simulink model "Queueing_system"  (R2023b)
settings: Solver=VariableStepAuto  StartTime=0.0  StopTime=100000.0  RelTol=1e-3
values from neighbouring files (symbols this model uses):
  m = 20    [Lab2_driver.m]
undefined symbols (not defined in the file or in its folder): entity, entitySys, n, ShowAttrib
settings Model: Creator=alberto  LastModifiedBy=alberto

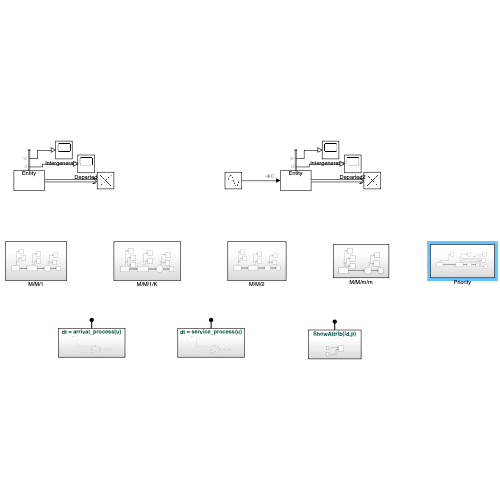
[thumbnail: Simulink's stored preview of the top-level diagram]
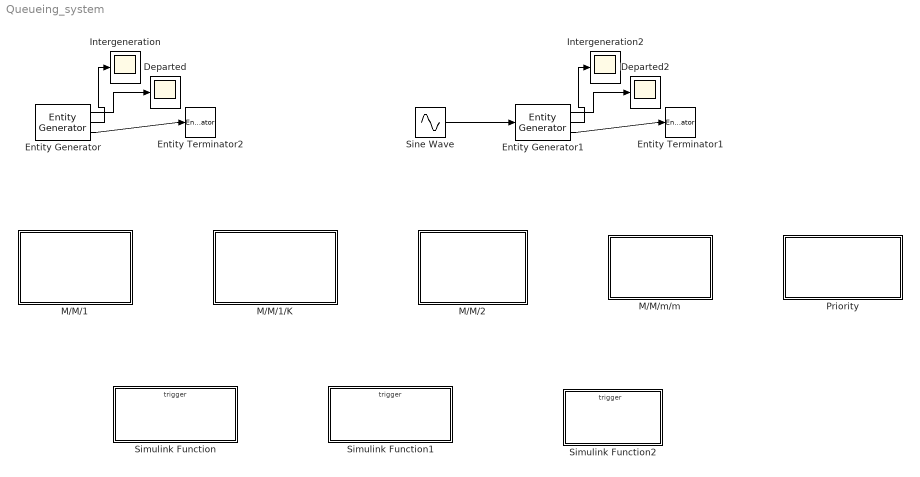
== system Queueing_system ==
  Departed : Scope
  Departed2 : Scope
  Entity Generator : EntityGenerator  OutputPortMessageModes=n,n,m  Period=0.5  IntergenerationTimeAction=dt = arrival_process(1/mG);  GenerateEntityAtSimulationStart=off  NumberEntitiesDeparted=on  AverageIntergenerationTime=on  EntityType=Structured  EntityTypeName=Entity
      settings: OutputPortMap=o0,o2,o3
  Entity Generator1 : EntityGenerator  OutputPortMessageModes=n,n,m  TimeSource=Signal port  Period=0.5  IntergenerationTimeAction=dt = arrival_process(1/mG);  GenerateEntityAtSimulationStart=off  NumberEntitiesDeparted=on  AverageIntergenerationTime=on  EntityType=Structured  EntityTypeName=Entity
      settings: InputPortMap=u1  OutputPortMap=o0,o2,o3
  Entity Terminator1 : EntityTerminator  InputPortMessageModes=m
  Entity Terminator2 : EntityTerminator  InputPortMessageModes=m
  Intergeneration : Scope
  Intergeneration2 : Scope
  M/M/1 : Subsystem
  M/M/1/K : Subsystem
  M/M/2 : Subsystem
  M/M/m/m : Subsystem
  Priority : Subsystem
  Simulink Function : Subsystem  TreatAsAtomicUnit=on
  Simulink Function1 : Subsystem  TreatAsAtomicUnit=on
  Simulink Function2 : Subsystem  TreatAsAtomicUnit=on
  Sine Wave : Sin  Bias=1.5  Frequency=2*pi  SampleTime=0
  wires:
  Sine Wave/1 -> Entity Generator1/1
  Entity Generator1/3 -> Entity Terminator1/1
  Entity Generator/3 -> Entity Terminator2/1
  Entity Generator/2 -> Intergeneration/1
  Entity Generator/1 -> Departed/1
  Entity Generator1/1 -> Departed2/1
  Entity Generator1/2 -> Intergeneration2/1

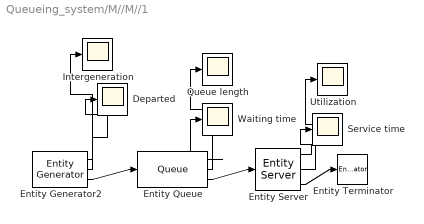
== system Queueing_system/M//M//1 ==
  Departed : Scope
  Entity Generator2 : EntityGenerator  OutputPortMessageModes=n,n,m  TimeSource=MATLAB action  Period=0.5  IntergenerationTimeAction=dt = arrival_process(1/mG);  GenerateEntityAtSimulationStart=off  NumberEntitiesDeparted=on  AverageIntergenerationTime=on  EntityType=Structured  EntityTypeName=Entity
      settings: OutputPortMap=o0,o2,o3
  Entity Queue : Queue  InputPortMessageModes=m  OutputPortMessageModes=n,n,m  Capacity=Inf  AverageWait=on  AverageQueueLength=on
      settings: OutputPortMap=o2,o3,o5
  Entity Server : EntityServer  InputPortMessageModes=m  OutputPortMessageModes=n,n,m  Capacity=1  ServiceTimeSource=MATLAB action  ServiceTimeAction=dt = service_process(1/mS);  AverageWait=on  Utilization=on
      settings: OutputPortMap=o4,o5,o9
  Entity Terminator : EntityTerminator  InputPortMessageModes=m
  Intergeneration : Scope
  Queue length : Scope
  Service time : Scope
  Utilization : Scope
  Waiting time : Scope
  wires:
  Entity Queue/1 -> Waiting time/1
  Entity Generator2/2 -> Intergeneration/1
  Entity Queue/3 -> Entity Server/1
  Entity Server/1 -> Service time/1
  Entity Generator2/3 -> Entity Queue/1
  Entity Server/2 -> Utilization/1
  Entity Generator2/1 -> Departed/1
  Entity Server/3 -> Entity Terminator/1
  Entity Queue/2 -> Queue length/1

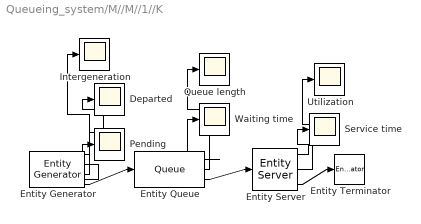
== system Queueing_system/M//M//1//K ==
  Departed : Scope
  Entity Generator : EntityGenerator  OutputPortMessageModes=n,n,n,m  TimeSource=MATLAB action  Period=0.5  IntergenerationTimeAction=dt = arrival_process(1/mG);  GenerateEntityAtSimulationStart=off  NumberEntitiesDeparted=on  PendingEntityInBlock=on  AverageIntergenerationTime=on  EntityType=Structured  EntityTypeName=Entity
      settings: OutputPortMap=o0,o1,o2,o3
  Entity Queue : Queue  InputPortMessageModes=m  OutputPortMessageModes=n,n,m  Capacity=K  AverageWait=on  AverageQueueLength=on
      settings: OutputPortMap=o2,o3,o5
  Entity Server : EntityServer  InputPortMessageModes=m  OutputPortMessageModes=n,n,m  Capacity=1  ServiceTimeSource=MATLAB action  ServiceTimeAction=dt = service_process(1/mS);  AverageWait=on  Utilization=on
      settings: OutputPortMap=o4,o5,o9
  Entity Terminator : EntityTerminator  InputPortMessageModes=m
  Intergeneration : Scope
  Pending : Scope
  Queue length : Scope
  Service time : Scope
  Utilization : Scope
  Waiting time : Scope
  wires:
  Entity Server/2 -> Utilization/1
  Entity Queue/2 -> Queue length/1
  Entity Queue/1 -> Waiting time/1
  Entity Queue/3 -> Entity Server/1
  Entity Generator/4 -> Entity Queue/1
  Entity Generator/3 -> Intergeneration/1
  Entity Generator/1 -> Departed/1
  Entity Generator/2 -> Pending/1
  Entity Server/1 -> Service time/1
  Entity Server/3 -> Entity Terminator/1

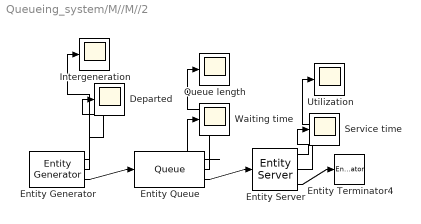
== system Queueing_system/M//M//2 ==
  Departed : Scope
  Entity Generator : EntityGenerator  OutputPortMessageModes=n,n,m  TimeSource=MATLAB action  Period=0.5  IntergenerationTimeAction=dt = arrival_process(1/mG);  GenerateEntityAtSimulationStart=off  NumberEntitiesDeparted=on  AverageIntergenerationTime=on  EntityType=Structured  EntityTypeName=Entity
      settings: OutputPortMap=o0,o2,o3
  Entity Queue : Queue  InputPortMessageModes=m  OutputPortMessageModes=n,n,m  Capacity=Inf  AverageWait=on  AverageQueueLength=on
      settings: OutputPortMap=o2,o3,o5
  Entity Server : EntityServer  InputPortMessageModes=m  OutputPortMessageModes=n,n,m  Capacity=2  ServiceTimeSource=MATLAB action  ServiceTimeAction=dt = service_process(1/mS);  AverageWait=on  Utilization=on
      settings: OutputPortMap=o4,o5,o9
  Entity Terminator4 : EntityTerminator  InputPortMessageModes=m
  Intergeneration : Scope
  Queue length : Scope
  Service time : Scope
  Utilization : Scope
  Waiting time : Scope
  wires:
  Entity Generator/2 -> Intergeneration/1
  Entity Queue/1 -> Waiting time/1
  Entity Server/1 -> Service time/1
  Entity Server/3 -> Entity Terminator4/1
  Entity Queue/2 -> Queue length/1
  Entity Queue/3 -> Entity Server/1
  Entity Server/2 -> Utilization/1
  Entity Generator/1 -> Departed/1
  Entity Generator/3 -> Entity Queue/1

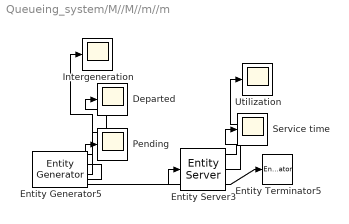
== system Queueing_system/M//M//m//m ==
  Departed : Scope
  Entity Generator5 : EntityGenerator  OutputPortMessageModes=n,n,n,m  TimeSource=MATLAB action  Period=0.5  IntergenerationTimeAction=dt = arrival_process(1/mG);  GenerateEntityAtSimulationStart=off  NumberEntitiesDeparted=on  PendingEntityInBlock=on  AverageIntergenerationTime=on  EntityType=Structured  EntityTypeName=Entity
      settings: OutputPortMap=o0,o1,o2,o3
  Entity Server3 : EntityServer  InputPortMessageModes=m  OutputPortMessageModes=n,n,m  Capacity=m  ServiceTimeSource=MATLAB action  ServiceTimeAction=dt = service_process(1/mS);  AverageWait=on  Utilization=on
      settings: OutputPortMap=o4,o5,o9
  Entity Terminator5 : EntityTerminator  InputPortMessageModes=m
  Intergeneration : Scope
  Pending : Scope
  Service time : Scope
  Utilization : Scope
  wires:
  Entity Generator5/3 -> Intergeneration/1
  Entity Server3/2 -> Utilization/1
  Entity Server3/1 -> Service time/1
  Entity Server3/3 -> Entity Terminator5/1
  Entity Generator5/2 -> Pending/1
  Entity Generator5/4 -> Entity Server3/1
  Entity Generator5/1 -> Departed/1

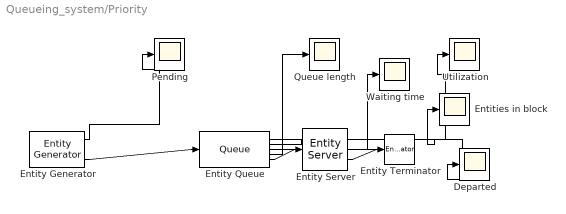
== system Queueing_system/Priority ==
  Departed : Scope
  Entities in block : Scope
  Entity Generator : EntityGenerator  OutputPortMessageModes=n,m  TimeSource=MATLAB action  Period=8  IntergenerationTimeAction=dt = arrival_process(1.5/mG);  GenerateEntityAtSimulationStart=off  GenerateAction=entity.MyPriority = randi(2);  AttributeName=MyPriority  AttributeInitialValue=0  PendingEntityInBlock=on  EntityType=Structured  EntityTypeName=Entity_p
      settings: OutputPortMap=o1,o3
  Entity Queue : Queue  InputPortMessageModes=m  OutputPortMessageModes=n,n,n,n,m  Capacity=Inf  QueueType=Priority  PrioritySource=MyPriority  ExitAction=ShowAttrib(entitySys.id, entity.MyPriority);  NumberEntitiesDeparted=on  NumberEntitiesInBlock=on  AverageWait=on  AverageQueueLength=on
      settings: OutputPortMap=o0,o1,o2,o3,o5
  Entity Server : EntityServer  InputPortMessageModes=m  OutputPortMessageModes=n,m  Capacity=1  ServiceTimeSource=MATLAB action  ServiceTimeAction=dt = service_process(1/mS);  Utilization=on
      settings: OutputPortMap=o5,o9
  Entity Terminator : EntityTerminator  InputPortMessageModes=m
  Pending : Scope
  Queue length : Scope
  Utilization : Scope
  Waiting time : Scope
  wires:
  Entity Queue/4 -> Queue length/1
  Entity Server/2 -> Entity Terminator/1
  Entity Generator/2 -> Entity Queue/1
  Entity Server/1 -> Utilization/1
  Entity Queue/1 -> Departed/1
  Entity Generator/1 -> Pending/1
  Entity Queue/5 -> Entity Server/1
  Entity Queue/3 -> Waiting time/1
  Entity Queue/2 -> Entities in block/1

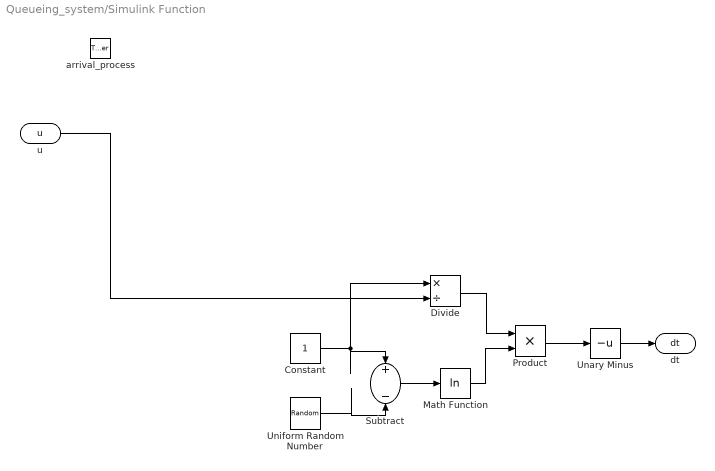
== system Queueing_system/Simulink Function ==
  arrival_process : TriggerPort  TriggerType=function-call  IsSimulinkFunction=on  FunctionName=arrival_process  FunctionVisibility=scoped  VariantControl=(inherit)
  Constant : Constant
  Divide : Product  Inputs=*/
  Math Function : Math  Operator=log
  Product : Product
  Subtract : Sum  Inputs=+-
  Unary Minus : UnaryMinus
  Uniform Random Number : UniformRandomNumber  Minimum=0  Seed=randi(3333333)
  u : ArgIn  DisableCoverage=on  ArgumentName=u
  dt : ArgOut  DisableCoverage=on  ArgumentName=dt
  wires:
  Product/1 -> Unary Minus/1
  Constant/1 -> Divide/1, Subtract/1
  u/1 -> Divide/2
  Uniform Random Number/1 -> Subtract/2
  Divide/1 -> Product/1
  Math Function/1 -> Product/2
  Subtract/1 -> Math Function/1
  Unary Minus/1 -> dt/1

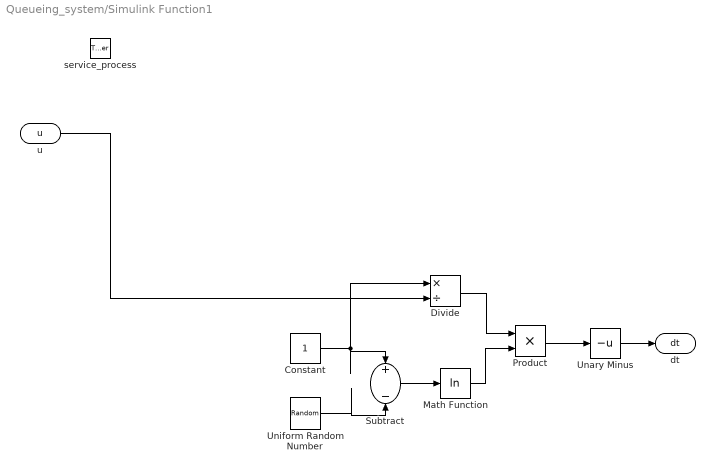
== system Queueing_system/Simulink Function1 ==
  service_process : TriggerPort  TriggerType=function-call  IsSimulinkFunction=on  FunctionName=service_process  FunctionVisibility=scoped  VariantControl=(inherit)
  Constant : Constant
  Divide : Product  Inputs=*/
  Math Function : Math  Operator=log
  Product : Product
  Subtract : Sum  Inputs=+-
  Unary Minus : UnaryMinus
  Uniform Random Number : UniformRandomNumber  Minimum=0  Seed=randi(7583)
  u : ArgIn  DisableCoverage=on  ArgumentName=u
  dt : ArgOut  DisableCoverage=on  ArgumentName=dt
  wires:
  Product/1 -> Unary Minus/1
  Constant/1 -> Divide/1, Subtract/1
  u/1 -> Divide/2
  Uniform Random Number/1 -> Subtract/2
  Divide/1 -> Product/1
  Math Function/1 -> Product/2
  Subtract/1 -> Math Function/1
  Unary Minus/1 -> dt/1

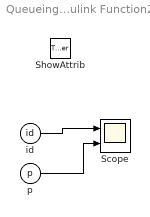
== system Queueing_system/Simulink Function2 ==
  ShowAttrib : TriggerPort  TriggerType=function-call  IsSimulinkFunction=on  FunctionName=ShowAttrib  FunctionVisibility=scoped  VariantControl=(inherit)
  Scope : Scope  NumInputPorts=2
  id : ArgIn  ArgumentName=id
  p : ArgIn  Port=2  ArgumentName=p
  wires:
  id/1 -> Scope/1
  p/1 -> Scope/2
